simulink library "MultiSourceEqBtc"  (R2022b)
settings: Solver=VariableStepAuto  StartTime=0.0  StopTime=10.0  RelTol=1e-3
undefined symbols (not defined in the file or in its folder): Row
libraries: TOP x3, TuneVar x3, FeaturePath x1, HandyTextFile x1, PoolIir x1, RTC x1
settings Model: Creator=kl13806  LastModifiedBy=yz1054030
settings SolverCC: AlgebraicLoopSolver=TrustRegion
settings DebuggingCC: UnconnectedInputMsg=warning  UnconnectedOutputMsg=warning  UnconnectedLineMsg=warning  SFMachineParentedDataDiag=warning
settings ModelReferenceCC: EnableRefExpFcnMdlSchedulingChecks=on
settings RTWCC: DLArmComputeVersion=19.05

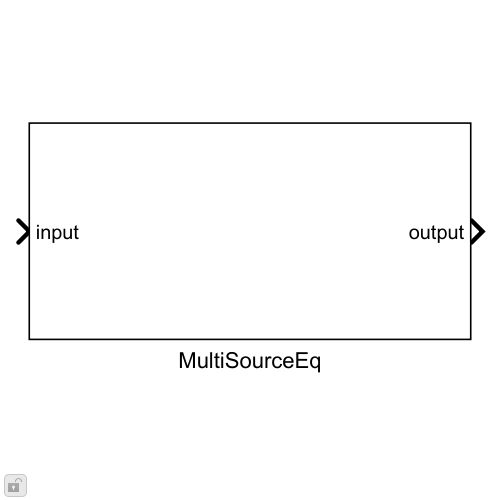
[thumbnail: Simulink's stored preview of the top-level diagram]
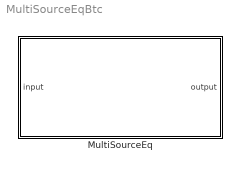
== system MultiSourceEqBtc ==
  MultiSourceEq : Subsystem  mask(Blocklib MultiSourceEq){Config=[], FeatureName=MultiSrcEQ}
      mask prompts: Config "MultiSourceEqConfig"; FeatureName "Feature path name:"
      mask init:
      | blkh=gcbh;
      | Config=BTConfig.Assert(blkh,Config);
      | 
      | Config.Validate();
      | BTConfig.InitSetFeatureIfPresent(blkh,'FeatureName');
      mask Callback Config: BTConfig.CallbackHideIfPresent(gcbh,{'FeatureName'});
      mask TypeOptions FeatureName: FeaturePath/FeatureName

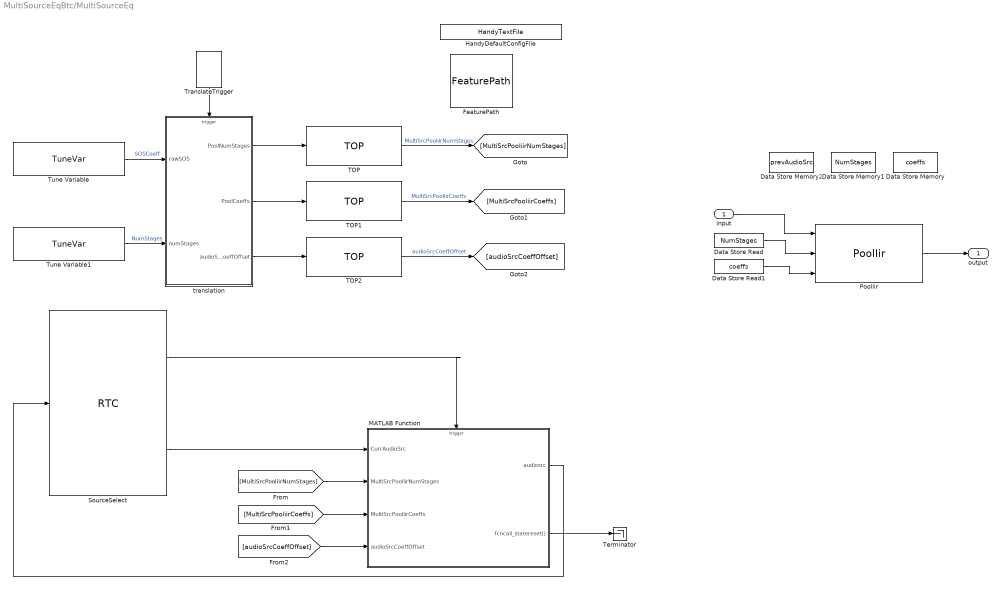
== system MultiSourceEqBtc/MultiSourceEq ==
  input : Inport
  Data Store Memory : DataStoreMemory  DataStoreName=coeffs  InitialValue=Config.InitialPoolSosCoeff  ShowAdditionalParam=off  OutDataTypeStr=single
  Data Store Memory1 : DataStoreMemory  DataStoreName=NumStages  InitialValue=Config.InitialPoolNumStages  ShowAdditionalParam=off  OutDataTypeStr=uint32
  Data Store Memory2 : DataStoreMemory  DataStoreName=prevAudioSrc  InitialValue=2^32  ShowAdditionalParam=off  OutDataTypeStr=uint32
  Data Store Read : DataStoreRead  DataStoreName=NumStages  IndexOptions=Index vector (dialog)  Indices=1  OutputSizes=1
  Data Store Read1 : DataStoreRead  DataStoreName=coeffs  IndexOptions=Index vector (dialog)  Indices=1  OutputSizes=1
  FeaturePath : FeaturePath/FeaturePath  FeatureName=MultiSrcEQ  IsGroup=off  GroupNumber=-1  IsModule=off  TriggerInit=[-410 -526 -315 -444]
      settings: SourceProductName=Bose Talaria
  HandyDefaultConfigFile : HandyTextFile/HandyTextFile  TemplateSource=Config  FileSuffix=Init  OpenDialogOnLoad=off  UseThisBlockName=off  AddGrandParentNamePrefix=off  TheDefaultText=|  ShowInLibBrowser=on
      | % $(FILENAME) Setup model parameters for each "Init" callback (e.g. update diagram)
      | sample_rate_in_hertz = 44100;
      | frame_size = 32;
      | sysin_channel_count = 2;
      settings: SourceProductName=Bose Talaria
  MATLAB Function : MATLAB Function  TreatAsAtomicUnit=on  mask{num_ent_audio_sources=Config.NumEntAudioSources, num_ent_channel=Config.NumEntChannel, num_stages_per_audio_source=Config.NumStagesPerAudioSource}
  PoolIir : PoolIir/PoolIir  Config=Config.PoolIir
  SourceSelect : RTC/RTC  REQ_Priority=RTC_Mask.NormalPriority  RequestAtInit=off  EnableRequest=on  REQElemName1=curAudioSrc  REQElemType1=uint32  REQElemWidth1=1  REQElemInitial1=[1]  REQElemType2=uint32  REQElemWidth2=1  REQElemInitial2=[]  REQElemType3=uint32  REQElemWidth3=1  REQElemInitial3=[]  REQElemType4=uint32  REQElemWidth4=1  REQElemInitial4=[]  REQElemType5=uint32  REQElemWidth5=1  REQElemInitial5=[]  REQElemType6=uint32  REQElemWidth6=1  REQElemInitial6=[]  REQElemType7=uint32  REQElemWidth7=1  REQElemInitial7=[]  REQElemType8=uint32  REQElemWidth8=1  REQElemInitial8=[]  REQElemType9=uint32  REQElemWidth9=1  REQElemInitial9=[]  REQElemType10=uint32  REQElemWidth10=1  REQElemInitial10=[]  EnableResponse=on  EnableRSP_StatusIn=off  RSPElemName1=curAudioSrc  RSPElemType1=uint32  RSPElemWidth1=1  RSPElemType2=uint32  RSPElemWidth2=1  RSPElemType3=uint32  RSPElemWidth3=1  RSPElemType4=uint32  RSPElemWidth4=1  RSPElemType5=uint32  RSPElemWidth5=1  RSPElemType6=uint32  RSPElemWidth6=1  RSPElemType7=uint32  RSPElemWidth7=1  RSPElemType8=uint32  RSPElemWidth8=1  RSPElemType9=uint32  RSPElemWidth9=1  RSPElemType10=uint32  RSPElemWidth10=1  EnableNotification=off  EnableNTF_PrepTrig=off  NTFElemType1=uint32  NTFElemWidth1=1  NTFElemType2=uint32  NTFElemWidth2=1  NTFElemType3=uint32  NTFElemWidth3=1  NTFElemType4=uint32  NTFElemWidth4=1  NTFElemType5=uint32  NTFElemWidth5=1  NTFElemType6=uint32  NTFElemWidth6=1  NTFElemType7=uint32  NTFElemWidth7=1  NTFElemType8=uint32  NTFElemWidth8=1  NTFElemType9=uint32  NTFElemWidth9=1  NTFElemType10=uint32  NTFElemWidth10=1  MaskMessageName=SourceSelect
      settings: SourceProductName=Bose Talaria
  TOP : TOP/TOP  TriggerInit=[-630 -415 -485 -355]  TopName=MultiSrcPooliirNumStages  DataType=uint32  BankNumber=0  PreOverlay=false  PostOverlay=false  Role=Automatic
      settings: SourceProductName=Bose Talaria
  TOP1 : TOP/TOP  TriggerInit=[-630 -330 -485 -270]  TopName=MultiSrcPooliirCoeffs  DataType=single  BankNumber=0  PreOverlay=false  PostOverlay=false  Role=Automatic
      settings: SourceProductName=Bose Talaria
  TOP2 : TOP/TOP  TriggerInit=[-630 -245 -485 -185]  TopName=audioSrcCoeffOffset  DataType=uint32  BankNumber=0  PreOverlay=false  PostOverlay=false  Role=Automatic
      settings: SourceProductName=Bose Talaria
  Terminator : Terminator
  TranslateTrigger : TuneVar/TranslateTrigger  TriggerInit=[-799 -530 -761 -475]
      settings: SourceProductName=Bose Talaria
  Tune Variable : TuneVar/TuneVar  TuneName=SOSCoeff  SpecifyMaxSize=on  VariableDim=1 (Row)  MaxSize=[Config.MaxNumEntInputStages 6]  TunabilityNumber=1  MinValue=[]  MaxValue=[]  TriggerInit=[-1080 -390 -910 -340]  MaskValue=Config.DefaultMultiSrcRawCoeffs
      settings: SourceProductName=Bose Talaria
  Tune Variable1 : TuneVar/TuneVar  TuneName=NumStages  SpecifyMaxSize=off  VariableDim=1 (Row)  MaxSize=[1 1]  TunabilityNumber=1  MinValue=[]  MaxValue=[]  TriggerInit=[-1080 -260 -910 -210]  MaskValue=Config.DefaultMultiSourceNumStages
      settings: SourceProductName=Bose Talaria
  translation : MATLAB Function  TreatAsAtomicUnit=on  mask{num_ent_channel=Config.NumEntChannel, num_ent_audio_sources=Config.NumEntAudioSources, max_num_ent_input_eq_stages=Config.MaxNumEntInputStages}
  output : Outport
  wires:
  PoolIir/1 -> output/1
  input/1 -> PoolIir/1
  Data Store Read/1 -> PoolIir/2
  Data Store Read1/1 -> PoolIir/3
  TOP2/1 -> [audioSrcCoeffOffset]  "audioSrcCoeffOffset"
  translation/3(audioSrcCoeffOffset) -> TOP2/1
  [audioSrcCoeffOffset] -> MATLAB Function/4(audioSrcCoeffOffset)
  MATLAB Function/1(audiosrc) -> SourceSelect/1
  [MultiSrcPooliirNumStages] -> MATLAB Function/2(MultiSrcPooliirNumStages)
  [MultiSrcPooliirCoeffs] -> MATLAB Function/3(MultiSrcPooliirCoeffs)
  TOP1/1 -> [MultiSrcPooliirCoeffs]  "MultiSrcPooliirCoeffs"
  TOP/1 -> [MultiSrcPooliirNumStages]  "MultiSrcPooliirNumStages"
  SourceSelect/1 -> MATLAB Function/Trigger
  SourceSelect/2 -> MATLAB Function/1(CurrAudioSrc)
  Tune Variable1/1 -> translation/2(numStages)  "NumStages"
  translation/2(PoolCoeffs) -> TOP1/1
  translation/1(PoolNumStages) -> TOP/1
  Tune Variable/1 -> translation/1(rawSOS)  "SOSCoeff"
  TranslateTrigger/1 -> translation/Trigger
  MATLAB Function/2(fcncall_statereset()) -> Terminator/1

== matlab function MultiSourceEqBtc/MultiSourceEq/MATLAB Function ==
  data: CurrAudioSrc input; MultiSrcPooliirNumStages input; audiosrc output; MultiSrcPooliirCoeffs input; audioSrcCoeffOffset input; prevAudioSrc data_store_memory; NumStages data_store_memory; coeffs data_store_memory; num_ent_audio_sources parameter; num_ent_channel parameter; num_stages_per_audio_source parameter
  events: trigger input FUNCTION_CALL_EVENT; fcncall_statereset output FUNCTION_CALL_EVENT
function audiosrc = MultiSourceEQConfigure(CurrAudioSrc,MultiSrcPooliirNumStages,MultiSrcPooliirCoeffs,...
                                           audioSrcCoeffOffset,num_ent_audio_sources,num_ent_channel,num_stages_per_audio_source)
    %#codegen
    %% datastore memory to control the audio processing logic:
    global prevAudioSrc;
    global NumStages;
    global coeffs;
    
    %% set the status to 0 to indicate the incorrect request is made
    %status = uint32(0);
    audiosrc = uint32(1);
    
    %% check appropriate audio source is set
    if((CurrAudioSrc > 0) && (CurrAudioSrc<=num_ent_audio_sources))
        
        %% check whether the previous audio source and current audio are different
        %% If the current audio is different, then following action are peformed:
        %%     * Reset the states of the pooliir filter
        %%     * Load the coefficient set of the requested the audio source
        %%     * Load the numStages for each channels for the selected source
        
        if (CurrAudioSrc ~= prevAudioSrc)
            %% function call to reset the filter states
            fcncall_statereset();
            %% Compute total coefficient should be loaded for the selected source
            totat_coeff_size = num_stages_per_audio_source * 4 + num_ent_channel;
            %% to overcome Dimension problem, defined coder.varsize
            pooliircoeffs = single(zeros(totat_coeff_size,1));
            start_idx = audioSrcCoeffOffset(CurrAudioSrc);
            end_idx = audioSrcCoeffOffset(CurrAudioSrc+1);
            pooliircoeffs(1:(end_idx-start_idx)) = MultiSrcPooliirCoeffs(start_idx:end_idx-1);
            %% Load the coeffcient
            coeffs = pooliircoeffs;
            %% to overcome Dimension problem, defined coder.varsize
            coder.varsize('stages');
            stagesoffset = (num_ent_channel*(CurrAudioSrc-1))+1;
            stages = MultiSrcPooliirNumStages(stagesoffset:stagesoffset+num_ent_channel-1);
            %% Load number of states per channel
            NumStages = stages(1:num_ent_channel);
            
            %% store the current audio src
            prevAudioSrc = CurrAudioSrc;
        end
        audiosrc = CurrAudioSrc;
    end

== matlab function MultiSourceEqBtc/MultiSourceEq/translation ==
  data: rawSOS input; numStages input; max_num_ent_input_eq_stages parameter; PoolNumStages output; PoolCoeffs output; num_ent_audio_sources parameter; num_ent_channel parameter; audioSrcCoeffOffset output
  events: trigger input FUNCTION_CALL_EVENT
function [PoolNumStages, PoolCoeffs,audioSrcCoeffOffset]  = MultiSrcpooliirTranslation(rawSOS, numStages,max_num_ent_input_eq_stages, num_ent_audio_sources, num_ent_channel)
    % Invoke pool iir translation function to compute num stages & coeffs
    [PoolNumStages, PoolCoeffs] = pooliirTranslationFcn(rawSOS, numStages,max_num_ent_input_eq_stages);
    audioSrcCoeffOffset = uint32(ones(1,num_ent_audio_sources+1));
    % compute the offset to fetch the correct coeffs for each source and 
    % for respective channels of the source
    for src = 1:num_ent_audio_sources
        offsetcount = uint32(0);
        for ch = 1:num_ent_channel
            offsetcount = offsetcount+(1+ 4*uint32(PoolNumStages(((src-1)*num_ent_channel)+ch)));
        end
        audioSrcCoeffOffset(src+1) = uint32(offsetcount+audioSrcCoeffOffset(src));
    end 
end
